simulink model "sys_dae_act_atk"  (R2021a)
settings: Solver=ode23t  StartTime=0.0  StopTime=30  RelTol=1e-3
settings Model: Creator=Suman  LastModifiedBy=Suman

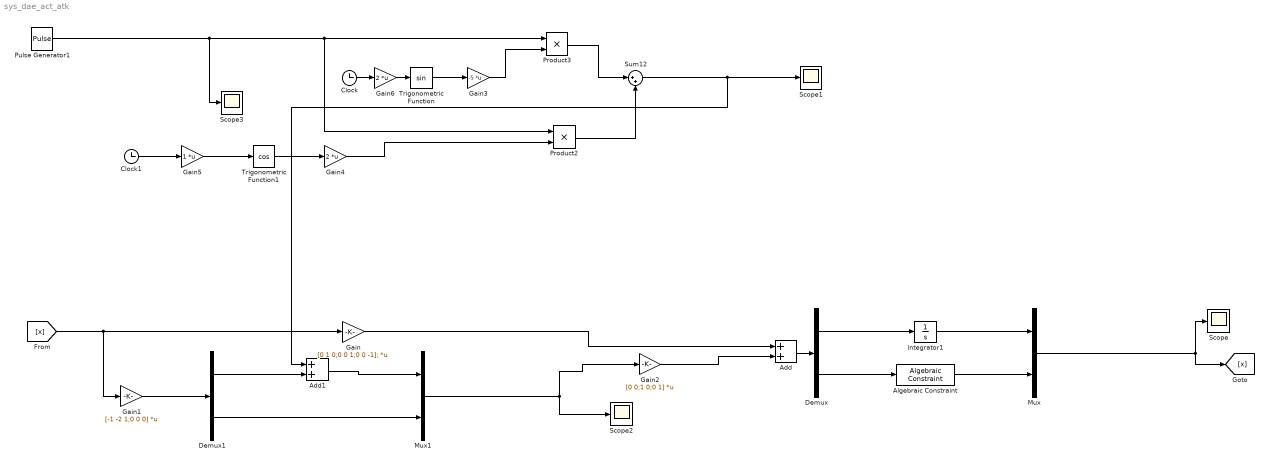
== system sys_dae_act_atk ==
  Add : Sum
  Add1 : Sum
  Algebraic Constraint : AlgebraicConstraint
  Clock : Clock
  Clock1 : Clock
  Demux : Demux  Outputs=2
  Demux1 : Demux  Outputs=2
  Gain : Gain  Gain=[0 1 0;0 0 1;0 0 -1];  Multiplication=Matrix(K*u) (u vector)
  Gain1 : Gain  Gain=[-1 -2 1;0 0 0]  Multiplication=Matrix(K*u) (u vector)
  Gain2 : Gain  Gain=[0 0;1 0;0 1]  Multiplication=Matrix(K*u) (u vector)
  Gain3 : Gain  Gain=-5  Multiplication=Matrix(K*u) (u vector)
  Gain4 : Gain  Gain=2  Multiplication=Matrix(K*u) (u vector)
  Gain5 : Gain  Multiplication=Matrix(K*u) (u vector)
  Gain6 : Gain  Gain=2  Multiplication=Matrix(K*u) (u vector)
  Integrator1 : Integrator  InitialCondition=[2;3]
  Mux : Mux  Inputs=2
  Mux1 : Mux  Inputs=2
  Product2 : Product
  Product3 : Product
  Pulse Generator1 : DiscretePulseGenerator  PulseType=Time based  Period=30  PulseWidth=10  PhaseDelay=10
  Scope{,1..3} (4 alike) : Scope
  Sum12 : Sum  Inputs=|++
  Trigonometric Function : Trigonometry
  Trigonometric Function1 : Trigonometry  Operator=cos
  wires:
  Demux/2 -> Algebraic Constraint/1
  Demux/1 -> Integrator1/1
  Integrator1/1 -> Mux/1
  Algebraic Constraint/1 -> Mux/2
  Mux/1 -> Scope/1, [x]
  Add/1 -> Demux/1
  Gain2/1 -> Add/2
  Gain/1 -> Add/1
  [x] -> Gain1/1, Gain/1
  Sum12/1 -> Add1/1, Scope1/1
  Product2/1 -> Sum12/2
  Product3/1 -> Sum12/1
  Clock/1 -> Gain6/1
  Clock1/1 -> Gain5/1
  Trigonometric Function1/1 -> Gain4/1
  Gain4/1 -> Product2/2
  Gain6/1 -> Trigonometric Function/1
  Trigonometric Function/1 -> Gain3/1
  Gain3/1 -> Product3/2
  Gain5/1 -> Trigonometric Function1/1
  Pulse Generator1/1 -> Scope3/1, Product2/1, Product3/1
  Mux1/1 -> Scope2/1, Gain2/1
  Gain1/1 -> Demux1/1
  Demux1/1 -> Add1/2
  Add1/1 -> Mux1/1
  Demux1/2 -> Mux1/2
